simulink model "Lab3_model_only"  (R2012b)
settings: Solver=ode45  StartTime=0.0  StopTime=500  RelTol=1e-3
settings Model: Creator=Viktor  LastModifiedBy=Viktor

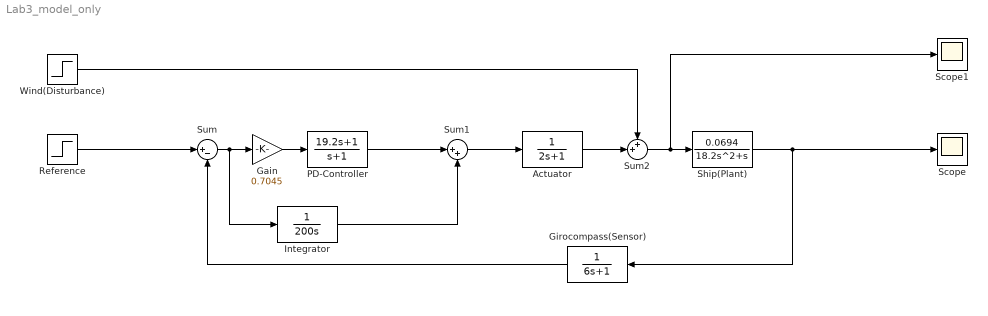
== system Lab3_model_only ==
  Actuator : TransferFcn  Denominator=[2 1]
  Gain : Gain  Gain=0.7045
  Girocompass(Sensor) : TransferFcn  Denominator=[6 1]
  Integrator : TransferFcn  Denominator=[200 0]
  PD-Controller : TransferFcn  Numerator=[19.2 1]  Denominator=[1 1]
  Reference : Step  Time=0  After=10  SampleTime=0
  Scope : Scope
  Scope1 : Scope
  Ship(Plant) : TransferFcn  Numerator=[0.0694]  Denominator=[18.2 1 0]
  Sum : Sum  Inputs=|+-
  Sum1 : Sum  Inputs=|++
  Sum2 : Sum  Inputs=++|
  Wind(Disturbance) : Step  Time=0  After=2  SampleTime=0
  wires:
  Ship(Plant)/1 -> Scope/1, Girocompass(Sensor)/1
  Girocompass(Sensor)/1 -> Sum/2
  Reference/1 -> Sum/1
  Gain/1 -> PD-Controller/1
  Sum/1 -> Integrator/1, Gain/1
  PD-Controller/1 -> Sum1/1
  Sum1/1 -> Actuator/1
  Integrator/1 -> Sum1/2
  Actuator/1 -> Sum2/2
  Sum2/1 -> Scope1/1, Ship(Plant)/1
  Wind(Disturbance)/1 -> Sum2/1
